simulink model "FIR_LMS_3_1"  (R2019b)
settings: Solver=FixedStepDiscrete  StartTime=0.0  StopTime=100e-6  RelTol=1e-3
libraries: xbsIndex_r4 x87
settings Model: Creator=blaisvin  LastModifiedBy=berniecl

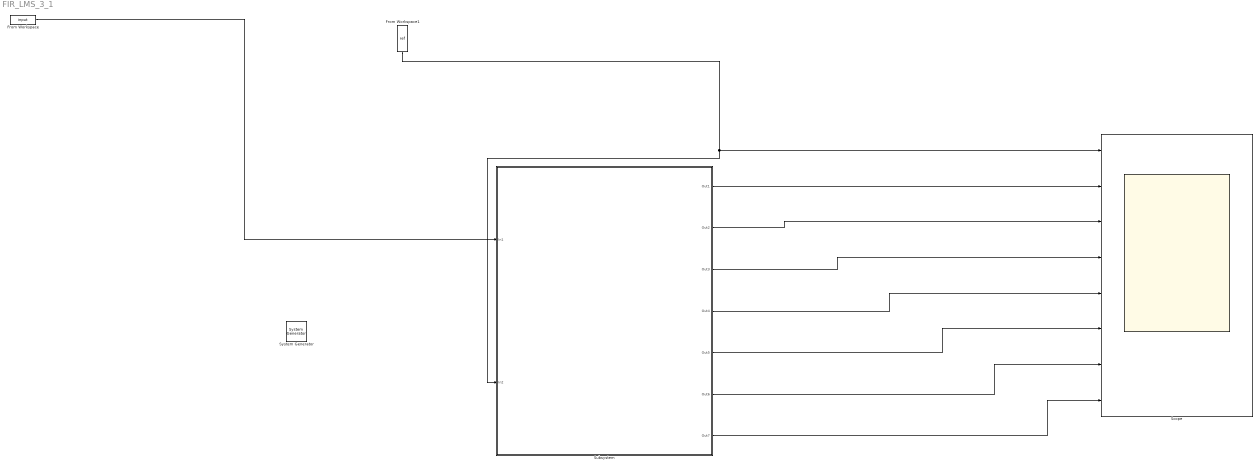
== system FIR_LMS_3_1 ==
  " System Generator" : xbsIndex_r4/ System Generator  Tag=genX  xilinxfamily=kintex7  part=xc7k325t  speed=-3  package=fbg676  synthesis_tool=Vivado  clock_wrapper=Clock Enables  directory=./netlist  proj_type=Vivado  Synth_file=Vivado Synthesis Defaults  Impl_file=Vivado Implementation Defaults  testbench=on  simulink_period=1/20e6  sysclk_period=50  dcm_input_clock_period=10  incr_netlist=off  trim_vbits=Everywhere in SubSystem  dbl_ovrd=According to Block Masks  core_generation=According to Block Masks  run_coregen=off  deprecated_control=off  eval_field=0  block_type=sysgen
  From Workspace : FromWorkspace  VariableName=input  SampleTime=0
  From Workspace1 : FromWorkspace  VariableName=ref  SampleTime=0
  Scope : Scope  NumInputPorts=8
  Subsystem : Subsystem
  wires:
  From Workspace1/1 -> Scope/1, Subsystem/2(In2)
  From Workspace/1 -> Subsystem/1(In1)
  Subsystem/1(Out1) -> Scope/2
  Subsystem/2(Out2) -> Scope/3
  Subsystem/3(Out3) -> Scope/4
  Subsystem/4(Out4) -> Scope/5
  Subsystem/5(Out5) -> Scope/6
  Subsystem/6(Out6) -> Scope/7
  Subsystem/7(Out7) -> Scope/8

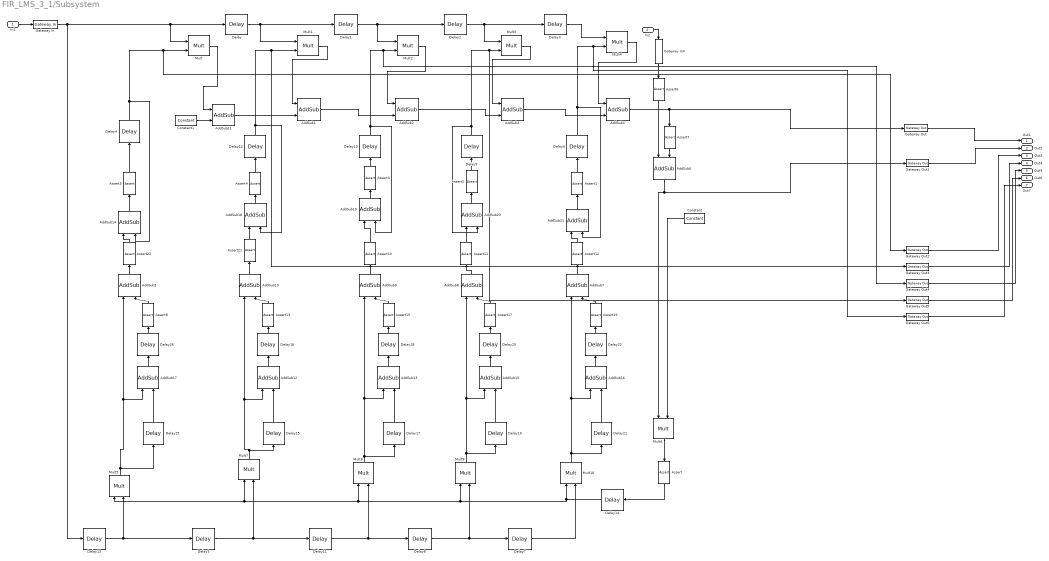
== system FIR_LMS_3_1/Subsystem ==
  In1 : Inport
  In2 : Inport  Port=2
  AddSub{1..3,11} (4 alike) : xbsIndex_r4/AddSub  mode=Addition  use_carryin=off  use_carryout=off  en=off  latency=0  precision=User Defined  arith_type=Unsigned  n_bits=16  bin_pt=14  quantization=Truncate  overflow=Wrap  use_behavioral_HDL=off  hw_selection=Fabric  pipelined=off  dbl_ovrd=off  block_type=addsub
  AddSub{4..5,7..10,12..21} (16 alike) : xbsIndex_r4/AddSub  mode=Addition  use_carryin=off  use_carryout=off  en=off  latency=0  precision=User Defined  arith_type="Signed  (2's comp)"  n_bits=16  bin_pt=14  quantization=Truncate  overflow=Wrap  use_behavioral_HDL=off  hw_selection=Fabric  pipelined=off  dbl_ovrd=off  block_type=addsub
  AddSub6 : xbsIndex_r4/AddSub  mode=Subtraction  use_carryin=off  use_carryout=off  en=off  latency=0  precision=User Defined  arith_type="Signed  (2's comp)"  n_bits=16  bin_pt=14  quantization=Truncate  overflow=Wrap  use_behavioral_HDL=off  hw_selection=Fabric  pipelined=off  dbl_ovrd=off  block_type=addsub
  Assert{,1..8,10..13,15,17,19,21..22} (18 alike) : xbsIndex_r4/Assert  assert_type=on  type_source=Explicitly  gui_display_data_type=Fixed-point  arith_type="Signed  (2's comp)"  n_bits=16  bin_pt=14  preci_type=Single  exp_width=8  frac_width=24  assert_rate=on  rate_source=Explicitly  period=1/20e6  output_port=on  block_type=assert
  Constant : xbsIndex_r4/Constant  const=0.25  gui_display_data_type=Fixed-point  arith_type=Signed (2's comp)  n_bits=16  bin_pt=14  preci_type=Single  exp_width=8  frac_width=24  explicit_period=off  period=1  equ=P=C  opselect=C  inp2=PCIN>>17  opr=+  inp1=P  carry=CIN  dbl_ovrd=off  block_type=constant
  Constant1 : xbsIndex_r4/Constant  const=0  gui_display_data_type=Fixed-point  arith_type=Signed (2's comp)  n_bits=16  bin_pt=14  preci_type=Single  exp_width=8  frac_width=24  explicit_period=off  period=1  equ=P=C  opselect=C  inp2=PCIN>>17  opr=+  inp1=P  carry=CIN  dbl_ovrd=off  block_type=constant
  Delay{,1..3,5,7..8,11,15..22,25..26} (18 alike) : xbsIndex_r4/Delay  rst=off  infoeditControl=Selection of Reset will increase slice count due to use of real FFs and instead of SRLs  en=off  latency=1  reg_retiming=off  dbl_ovrd=off  block_type=delay
  Delay{4,6,9..10,12} (5 alike) : xbsIndex_r4/Delay  rst=off  infoeditControl=Selection of Reset will increase slice count due to use of real FFs and instead of SRLs  en=off  latency=3  reg_retiming=off  dbl_ovrd=off  block_type=delay
  Delay13 : xbsIndex_r4/Delay  rst=off  infoeditControl=Selection of Reset will increase slice count due to use of real FFs and instead of SRLs  en=off  latency=5  reg_retiming=off  dbl_ovrd=off  block_type=delay
  Delay14 : xbsIndex_r4/Delay  rst=off  infoeditControl=Selection of Reset will increase slice count due to use of real FFs and instead of SRLs  en=off  latency=5  reg_retiming=off  dbl_ovrd=off  block_type=delay
  Gateway In : xbsIndex_r4/Gateway In  gui_display_data_type=Fixed-point  arith_type="Signed  (2's comp)"  n_bits=16  bin_pt=14  preci_type=Single  exp_width=8  frac_width=24  rows=1  columns=1  quantization="Round  (unbiased: +/- Inf)"  overflow=Saturate  period=1/20e6  UseAsADC=off  ADCChannel='1'  interface=None  automatic_assignment=on  address_offset=hex2dec('00')  intf_name=''  intf_description=''  default_value=0  timing_constraint=None  locs_specified=off  LOCs={}  io_standard={}  inherit_from_input=off  hdl_port=on  dbl_ovrd=off  block_type=gatewayin
  Gateway In4 : xbsIndex_r4/Gateway In  gui_display_data_type=Fixed-point  arith_type="Signed  (2's comp)"  n_bits=16  bin_pt=14  preci_type=Single  exp_width=8  frac_width=24  rows=1  columns=1  quantization="Round  (unbiased: +/- Inf)"  overflow=Saturate  period=1/20e6  UseAsADC=off  ADCChannel='1'  interface=None  automatic_assignment=on  address_offset=hex2dec('00')  intf_name=''  intf_description=''  default_value=0  timing_constraint=None  locs_specified=off  LOCs={}  io_standard={}  inherit_from_input=off  hdl_port=on  dbl_ovrd=off  block_type=gatewayin
  Gateway Out{,1..6} (7 alike) : xbsIndex_r4/Gateway Out  inherit_from_input=off  hdl_port=on  rows=1  columns=1  UseAsDAC=off  DACChannel='1'  interface=None  automatic_assignment=on  address_offset=hex2dec('00')  intf_name=''  intf_description=''  timing_constraint=None  locs_specified=off  LOCs={}  io_standard={}  block_type=gatewayout
  Mult{,1..10} (11 alike) : xbsIndex_r4/Mult  precision=User Defined  arith_type="Signed  (2's comp)"  n_bits=16  bin_pt=14  quantization=Truncate  overflow=Wrap  en=off  latency=0  use_behavioral_HDL=off  opt=Speed  use_embedded=on  optimum_pipeline=off  pipeline=on  dbl_ovrd=off  use_rpm=on  placement_style=Triangular  block_type=mult
  Out1 : Outport
  Out2 : Outport  Port=2
  Out3 : Outport  Port=3
  Out4 : Outport  Port=4
  Out5 : Outport  Port=5
  Out6 : Outport  Port=6
  Out7 : Outport  Port=7
  wires:
  Assert17/1 -> AddSub8/2
  Assert2/1 -> Delay9/1
  Delay22/1 -> Assert19/1
  Assert4/1 -> Delay12/1
  Gateway In/1 -> Delay13/1, Mult/1, Delay/1
  Delay17/1 -> AddSub13/2
  AddSub9/1 -> Assert10/1
  Delay10/1 -> AddSub19/2, Gateway Out4/1, Mult2/2
  Delay12/1 -> Gateway Out3/1, Mult1/2, AddSub18/2
  Delay6/1 -> AddSub21/2, Gateway Out6/1, Mult4/2
  Mult5/1 -> Delay25/1, AddSub17/1, AddSub5/1
  AddSub20/1 -> Assert2/1
  Assert21/1 -> AddSub18/1
  Delay2/1 -> Delay3/1, Mult3/1
  In1/1 -> Gateway In/1
  AddSub21/1 -> Assert1/1
  AddSub17/1 -> Delay26/1
  Assert10/1 -> AddSub19/1
  Delay7/1 -> Mult10/2
  Gateway In4/1 -> Assert6/1
  AddSub8/1 -> Assert11/1
  AddSub7/1 -> Assert12/1
  Delay16/1 -> Assert13/1
  Delay20/1 -> Assert17/1
  Mult/1 -> AddSub11/1
  AddSub12/1 -> Delay16/1
  AddSub15/1 -> Delay20/1
  Mult1/1 -> AddSub1/1
  Mult2/1 -> AddSub2/1
  Assert19/1 -> AddSub7/2
  Assert12/1 -> AddSub21/1
  Mult6/1 -> Assert/1
  Assert13/1 -> AddSub10/2
  Assert11/1 -> AddSub20/1
  Delay15/1 -> AddSub12/2
  Delay9/1 -> AddSub20/2, Gateway Out5/1, Mult3/2
  AddSub2/1 -> AddSub3/2
  Assert8/1 -> AddSub5/2
  AddSub14/1 -> Assert5/1
  AddSub10/1 -> Assert21/1
  AddSub16/1 -> Delay22/1
  Mult7/1 -> Delay15/1, AddSub10/1, AddSub12/1
  Assert6/1 -> AddSub6/1
  AddSub13/1 -> Delay18/1
  Assert15/1 -> AddSub9/2
  Assert22/1 -> AddSub14/1
  AddSub19/1 -> Assert3/1
  Delay21/1 -> AddSub16/2
  Mult8/1 -> AddSub13/1, AddSub9/1, Delay17/1
  Delay25/1 -> AddSub17/2
  Delay5/1 -> Delay11/1, Mult7/2
  Assert3/1 -> Delay10/1
  AddSub6/1 -> Gateway Out1/1, Mult6/1
  Mult9/1 -> Delay19/1, AddSub8/1, AddSub15/1
  Delay4/1 -> AddSub14/2, Gateway Out2/1, Mult/2
  AddSub5/1 -> Assert22/1
  Delay18/1 -> Assert15/1
  Delay26/1 -> Assert8/1
  AddSub1/1 -> AddSub2/2
  Assert5/1 -> Delay4/1
  Delay19/1 -> AddSub15/2
  AddSub11/1 -> AddSub1/2
  Assert/1 -> Delay14/1
  Mult10/1 -> Delay21/1, AddSub7/1, AddSub16/1
  Constant1/1 -> AddSub11/2
  Delay3/1 -> Mult4/1
  Mult4/1 -> AddSub4/1
  Gateway Out1/1 -> Out2/1
  Delay11/1 -> Delay8/1, Mult8/2
  Mult3/1 -> AddSub3/1
  Delay/1 -> Mult1/1, Delay1/1
  Delay8/1 -> Delay7/1, Mult9/2
  AddSub3/1 -> AddSub4/2
  Delay1/1 -> Mult2/1, Delay2/1
  AddSub4/1 -> Assert7/1, Gateway Out/1
  Constant/1 -> Mult6/2
  Delay14/1 -> Mult5/1, Mult7/1, Mult8/1, Mult9/1, Mult10/1
  Delay13/1 -> Delay5/1, Mult5/2
  AddSub18/1 -> Assert4/1
  Assert7/1 -> AddSub6/2
  Assert1/1 -> Delay6/1
  Gateway Out5/1 -> Out6/1
  Gateway Out4/1 -> Out5/1
  Gateway Out/1 -> Out1/1
  In2/1 -> Gateway In4/1
  Gateway Out6/1 -> Out7/1
  Gateway Out3/1 -> Out4/1
  Gateway Out2/1 -> Out3/1
